simulink library "qlib"  (Simulink 7.0)
libraries: qlib x9, simulink x4
Description:
  | Quaternion Library for Simulink
  |   Version 1.5 (JASP) 20-Jul-2009
  |   ========================================================================
  |   Copyright (c) 2000-2009, Jay A. St. Pierre.  All rights reserved.
  |   This software is licensed under the terms of the BSD license.
  |   See the file license.txt that came with the software for more details.
  |   ========================================================================
  | 
  |   This is a library of blocks that allows manipulation of quaternions.
  | 
  |   The available blocks are:
  | 
  |     Quaternion Normalize
  |     Quaternion Conjugate
  |     Quaternion Multiply
  | 
  |     Quaternion Propagation
  |     Quaternion Vector Transform
  |     Quaternion Vector Rotation
  | 
  |     Quaternion Decomposition
  |     Quaternion to DCM
  |     DCM to Quaternion
  | 
  |   For purposes of this library, a quaternion, q, is just a four element
  |   vector where q(1:3) is the "imaginary" or "vector" portion of the
  |   hypercomplex number, and q(4) is the "real" or "scalar" portion.
  |   Consequently, if q represents a rotation, then:
  | 
  |     q(1) = v1*sin(phi/2)
  |     q(2) = v2*sin(phi/2)
  |     q(3) = v3*sin(phi/2)
  |     q(4) =    cos(phi/2)
  | 
  |   where phi is the amount of rotation about the unit vector [v1 v2 v3].
  | 
  |   IMPORTANT NOTE: For purposes of quaternion/DCM equivalence, the
  |   relationship is chosen to be:
  | 
  |      R v = q* v q
  | 
  |   Therefore a "transform" is (q* v q) and a "rotation" is (q v q*). This
  |   follows the convention used in "Spacecraft Attitude Determination and
  |   Control", edited by James R. Wertz, Copyright 1978.  Note that many
  |   recent uses of quaternions choose the opposite convention (the "left"
  |   quaternion being the equivalent), including many computer graphics
  |   libraries.
  | 
  |   See also QUATERNIONS, the quaternion manipulation toolbox for the
  |   MATLAB command line.  RM2MAT and MAT2RM are also useful for handling
  |   row-major form matrices, and can be found in the Matrix Library for
  |   Simulink.
settings Model: Creator=stpierre  LastModifiedBy=stpierre  ExtModeAutoUpdateStatusClock=off

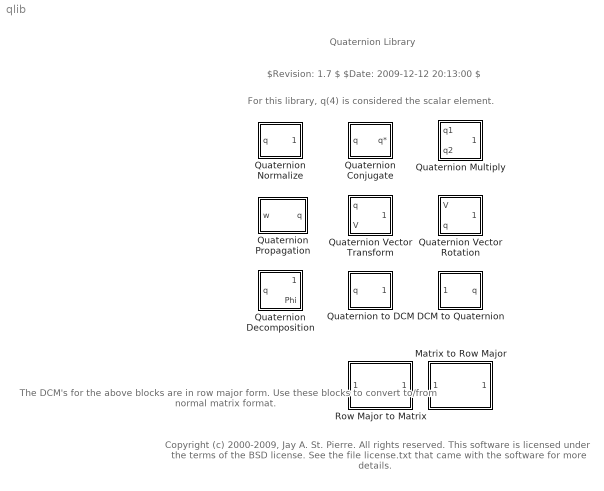
== system qlib ==
  note: Quaternion Library
  note: $Revision: 1.7 $
      | $Date: 2009-12-12 20:13:00 $
  note: For this library, q(4) is considered the scalar element.
  note: Copyright (c) 2000-2009, Jay A. St. Pierre.  All rights reserved.
      | This software is licensed under the terms of the BSD license.
      | See the file license.txt that came with the software for more details.
  note: The DCM's for the
      | above blocks are in
      | row major form.  Use
      | these blocks to convert
      | to/from normal matrix
      | format.
  DCM to Quaternion : Subsystem
      mask Type: DCM to Quaternion
      mask Description:
      | Converts a direction cosine matrix (DCM) to a quaternion that would perform the equivalent vector transformation, i.e., q*vq = Rv, where R is the DCM, v is a vector, and q is the quaternion.
      | 
      | Note that for purposes of quaternion-vector multiplication, a vector is treated as a quaterion with a scalar element of zero.
  Matrix to Row Major : Subsystem
      mask Type: Matrix to Row Major
      mask Description: Converts a matrix to row major vector form.
      mask Display: fprintf('Matrix to\nRow Major');
  Quaternion Conjugate : Subsystem
      mask Type: Quaternion Conjugate
      mask Description: q* = [ -q(1)  -q(2)  -q(3)  q(4) ]
      mask Display: disp('q*')
  Quaternion Decomposition : Subsystem
      mask Type: Quaternion Decomposition
      mask Description:
      | Breaks down a quaternion into its unit vector and total rotation angle about that vector.  If the components of the quaternion are denoted:
      | 
      |      q = [ q(1)  q(2)  q(3)  q(4) ]
      | 
      | Then:
      | 
      |      q(1) = v1 sin(phi/2)
      |      q(2) = v2 sin(phi/2)
      |      q(3) = v3 sin(phi/2)
      |      q(4) = cos(phi/2)
      | 
      | Where phi is the amount of rotation about the unit vector [ v1  v2  v3 ].
  Quaternion Multiply : Subsystem
      mask Type: Quaternion Multiply
      mask Description: Multiplies input quaternions: qout = (q1)(q2)
  Quaternion Normalize : Subsystem  mask(Quaternion Normalize){}
      mask help: qout = q/sqrt(q(1)^2+q(2)^2+q(3)^2+q(4)^2)
      mask init:
      | pos = get_param(gcb, 'Position');
      | width = pos(3) - pos(1); height = pos(4) - pos(2);
      | fontsize = get_param(gcb, 'fontsize');
      | if fontsize==-1, scale=1; else scale=fontsize/10; end
      mask Display:
      | text(width/2-scale*3, (height/2+scale*10), 'q')
      | text(width/2-scale*8, (height/2-scale*6), '||q||')
      | plot([width/2-scale*10 width/2+scale*10], height/2*[1 1])
  Quaternion Propagation : Subsystem  mask(Quaternion Propagation){q0=[0 0 0 1]}
      mask help:
      | Integrates dq/dt to propagate a quaternion, where:
      |
      |     dq/dt = (1/2) (q) ([w 0])
      |
      | and the product (q)([w 0]) is calculated as a quaternion multiplication.
      |
      | The input rates, w, are inertial, but written in the body frame coordinates.  The quaternion indicates the orientation of the body frame with respect to the inertial frame.  The initlal quaternion, q0, must be specfied below.
      |
      | The quaternion is renormalized at each iteration.
      mask init:
      | pos = get_param(gcb, 'Position');
      | width = pos(3) - pos(1); height = pos(4) - pos(2);
      | fontsize = get_param(gcb, 'fontsize');
      | if fontsize==-1, scale=1; else scale=fontsize/10; end
      | 
      | t1=-pi/2:(pi/2)/20:0; t2=pi:-(pi/2)/20:(pi/2);
      | x=[cos(t1)  cos(t2)+2]; y=[sin(t1)+1  sin(t2)+4];
      | 
      | ny=0.9*y/max(y)*scale;
      | nx=0.9*x/max(y)*scale;
      | 
      | s=20;
      | sy=s*(ny - max(ny)/2) + height/2;
      | sx=s*nx + width/2 - 15*scale;
      | 
      | t=0:2*pi/100:2*pi;
      | a=1;
      | tx=a*cos(t)+width/2-5*scale; ty=a*sin(t)+height/2+4*scale;
      mask Display:
      | plot(sx,sy);
      | text(width/2-7*scale, height/2, 'q dt');
      | plot(tx,ty)
  Quaternion Vector Rotation : Subsystem
      mask Type: Quaternion Vector Rotation
      mask Description:
      | Rotates a vector using a quaternion:
      | 
      |     vout = (q)(v)(q*)
      | 
      | The first input is the vector, the second input is the quaternion.
      | 
      | Note that for purposes of quaternion-vector multiplication, a vector is treated as a quaterion with a scalar element of zero.
  Quaternion Vector Transform : Subsystem
      mask Type: Quaternion Vector Transform
      mask Description:
      | Transforms a vector using a quaternion:
      | 
      |     vout = (q*)(v)(q)
      | 
      | The first input is the quaternion, the second input is the vector.
      | 
      | Note that for purposes of quaternion-vector multiplication, a vector is treated as a quaterion with a scalar element of zero.
  Quaternion to DCM : Subsystem
      mask Type: Quaternion to DCM
      mask Description:
      | Converts a quaternion to the direction cosine matrix (DCM) that would perform the equivalent vector transformation, i.e., Rv = q*vq, where R is the DCM, v is a vector, and q is the quaternion.
      | 
      | Note that for purposes of quaternion-vector multiplication, a vector is treated as a quaterion with a scalar element of zero.
  Row Major to Matrix : Subsystem  mask(Row Major to Matrix){rows=3, columns=3}
      mask help: Converts a row major representation of a matrix to a normal matrix.
      mask Display:
      | fprintf('Row Major\nto Matrix\n')
      | text(1, 0, ...
      |     sprintf('%dx%d', rows, columns), ...
      |     'HorizontalAlignment', 'Right', ...
      |     'VerticalAlignment', 'Bottom');

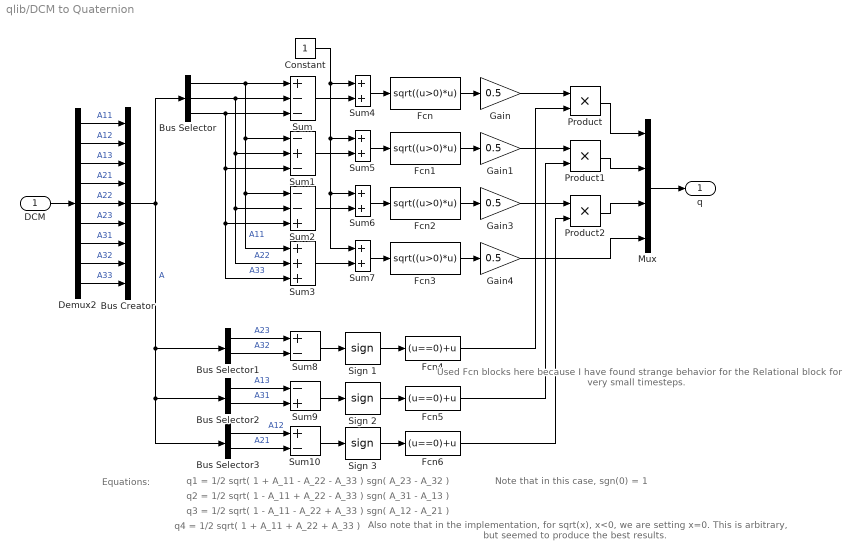
== system qlib/DCM to Quaternion ==
  note: Used Fcn blocks here because
      | I have found strange behavior
      | for the Relational block for
      | very small timesteps.
  note: q1 = 1/2 sqrt( 1 + A_11 - A_22 - A_33 ) sgn( A_23 - A_32 )
  note: q2 = 1/2 sqrt( 1 - A_11 + A_22 - A_33 ) sgn( A_31 - A_13 )
  note: q3 = 1/2 sqrt( 1 - A_11 - A_22 + A_33 ) sgn( A_12 - A_21 )
  note: q4 = 1/2 sqrt( 1 + A_11 + A_22 + A_33 )
  note: Equations:
  note: Note that in this case, sgn(0) = 1
  note: Also note that in the implementation,
      | for sqrt(x), x<0, we are setting x=0.
      | This is arbitrary, but seemed to produce
      | the best results.
  DCM : Inport  PortDimensions=9
  Bus Creator : BusCreator  Inputs=9
  Bus Selector : BusSelector  OutputSignals=A11,A22,A33
  Bus Selector1 : BusSelector  OutputSignals=A23,A32
  Bus Selector2 : BusSelector  OutputSignals=A13,A31
  Bus Selector3 : BusSelector  OutputSignals=A12,A21
  Constant : Constant
  Demux2 : Demux  Outputs=9
  Fcn{,1..3} (4 alike) : Fcn  Expr=sqrt((u>0)*u)
  Fcn4 : Fcn  Expr=(u==0)+u
  Fcn5 : Fcn  Expr=(u==0)+u
  Fcn6 : Fcn  Expr=(u==0)+u
  Gain{,1,3..4} (4 alike) : Gain  Gain=0.5  SaturateOnIntegerOverflow=on
  Mux : Mux
  Product : Product  SaturateOnIntegerOverflow=on  RndMeth=Zero  InputSameDT=on
  Product1 : Product  SaturateOnIntegerOverflow=on  RndMeth=Zero  InputSameDT=on
  Product2 : Product  SaturateOnIntegerOverflow=on  RndMeth=Zero  InputSameDT=on
  Sign 1 : Signum
  Sign 2 : Signum
  Sign 3 : Signum
  Sum : Sum  Inputs=+--  SaturateOnIntegerOverflow=on  InputSameDT=on
  Sum1 : Sum  Inputs=-+-  SaturateOnIntegerOverflow=on  InputSameDT=on
  Sum10 : Sum  Inputs=+-  SaturateOnIntegerOverflow=on  InputSameDT=on
  Sum2 : Sum  Inputs=--+  SaturateOnIntegerOverflow=on  InputSameDT=on
  Sum3 : Sum  Inputs=+++  SaturateOnIntegerOverflow=on  InputSameDT=on
  Sum{4..7} (4 alike) : Sum  SaturateOnIntegerOverflow=on  InputSameDT=on
  Sum8 : Sum  Inputs=+-  SaturateOnIntegerOverflow=on  InputSameDT=on
  Sum9 : Sum  Inputs=-+  SaturateOnIntegerOverflow=on  InputSameDT=on
  q : Outport  InitialOutput=[0 0 0 1]
  wires:
  Sum/1 -> Sum4/2
  Sum1/1 -> Sum5/2
  Constant/1 -> Sum4/1, Sum5/1, Sum6/1, Sum7/1
  Sum4/1 -> Fcn/1
  Sum3/1 -> Sum7/2
  Sum2/1 -> Sum6/2
  Gain/1 -> Product/1
  Gain1/1 -> Product1/1
  Gain3/1 -> Product2/1
  Sum5/1 -> Fcn1/1
  Sum6/1 -> Fcn2/1
  Sum7/1 -> Fcn3/1
  Fcn/1 -> Gain/1
  Fcn1/1 -> Gain1/1
  Fcn3/1 -> Gain4/1
  Fcn2/1 -> Gain3/1
  Sum8/1 -> Sign 1/1
  Fcn4/1 -> Product/2
  Sign 1/1 -> Fcn4/1
  Sum9/1 -> Sign 2/1
  Fcn5/1 -> Product1/2
  Sign 2/1 -> Fcn5/1
  Sum10/1 -> Sign 3/1
  Fcn6/1 -> Product2/2
  Sign 3/1 -> Fcn6/1
  Bus Selector1/1 -> Sum8/1  "A23"
  Bus Selector1/2 -> Sum8/2  "A32"
  Bus Selector/2 -> Sum/2, Sum1/2, Sum3/2, Sum2/2  "A22"
  Bus Selector/1 -> Sum/1, Sum1/1, Sum2/1, Sum3/1  "A11"
  Bus Selector/3 -> Sum/3, Sum1/3, Sum3/3, Sum2/3  "A33"
  Bus Selector2/1 -> Sum9/1  "A13"
  Bus Selector2/2 -> Sum9/2  "A31"
  Bus Selector3/2 -> Sum10/2  "A21"
  Bus Selector3/1 -> Sum10/1  "A12"
  Demux2/1 -> Bus Creator/1  "A11"
  Demux2/2 -> Bus Creator/2  "A12"
  Demux2/3 -> Bus Creator/3  "A13"
  Demux2/4 -> Bus Creator/4  "A21"
  Demux2/5 -> Bus Creator/5  "A22"
  Demux2/6 -> Bus Creator/6  "A23"
  Demux2/7 -> Bus Creator/7  "A31"
  Demux2/8 -> Bus Creator/8  "A32"
  Demux2/9 -> Bus Creator/9  "A33"
  DCM/1 -> Demux2/1
  Bus Creator/1 -> Bus Selector/1, Bus Selector1/1, Bus Selector2/1, Bus Selector3/1  "A"
  Product/1 -> Mux/1
  Product1/1 -> Mux/2
  Product2/1 -> Mux/3
  Gain4/1 -> Mux/4
  Mux/1 -> q/1

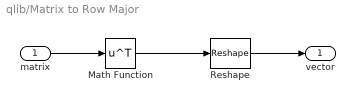
== system qlib/Matrix to Row Major ==
  matrix : Inport
  Math Function : Math  Operator=transpose  OutDataType=sfix(16)  OutScaling=2^0  SaturateOnIntegerOverflow=on
      settings: AttributesFormatString=%<Operator>
  Reshape : Reshape  OutputDimensions=[3, 3]
      settings: AttributesFormatString=Output: %<OutputDimensionality>
  vector : Outport
  wires:
  Math Function/1 -> Reshape/1
  matrix/1 -> Math Function/1
  Reshape/1 -> vector/1

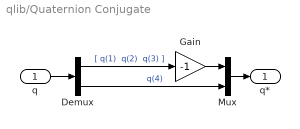
== system qlib/Quaternion Conjugate ==
  q : Inport  PortDimensions=4
  Demux : Demux  Outputs=[3 1]
  Gain : Gain  Gain=-1  SaturateOnIntegerOverflow=on
  Mux : Mux  Inputs=2
  q* : Outport  InitialOutput=0
  wires:
  q/1 -> Demux/1
  Demux/1 -> Gain/1  "[ q(1)  q(2)  q(3) ]"
  Gain/1 -> Mux/1
  Demux/2 -> Mux/2  "q(4)"
  Mux/1 -> q*/1

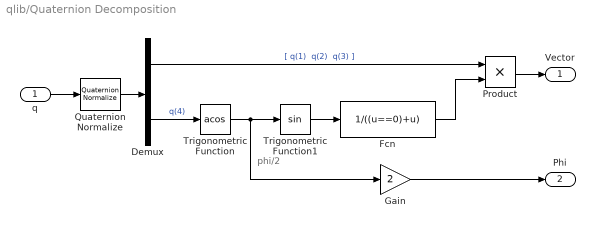
== system qlib/Quaternion Decomposition ==
  note: phi/2
  q : Inport  PortDimensions=4
  Demux : Demux  Outputs=[3 1]
  Fcn : Fcn  Expr=1/((u==0)+u)
  Gain : Gain  Gain=2  SaturateOnIntegerOverflow=on
  Product : Product  SaturateOnIntegerOverflow=on  RndMeth=Zero  InputSameDT=on
  Quaternion Normalize : qlib/Quaternion Normalize
  Trigonometric Function : Trigonometry  Operator=acos
  Trigonometric Function1 : Trigonometry
  Vector : Outport  InitialOutput=0
  Phi : Outport  Port=2  InitialOutput=0
  wires:
  Quaternion Normalize/1 -> Demux/1
  Demux/1 -> Product/1  "[ q(1)  q(2)  q(3) ]"
  Demux/2 -> Trigonometric Function/1  "q(4)"
  Trigonometric Function1/1 -> Fcn/1
  Trigonometric Function/1 -> Trigonometric Function1/1, Gain/1
  Gain/1 -> Phi/1
  q/1 -> Quaternion Normalize/1
  Product/1 -> Vector/1
  Fcn/1 -> Product/2

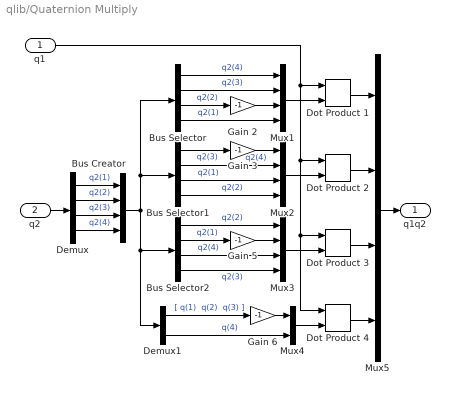
== system qlib/Quaternion Multiply ==
  q1 : Inport  PortDimensions=4
  q2 : Inport  Port=2  PortDimensions=4
  Bus Creator : BusCreator
  Bus Selector : BusSelector  OutputSignals=q2(4),q2(3),q2(2),q2(1)
  Bus Selector1 : BusSelector  OutputSignals=q2(3),q2(4),q2(1),q2(2)
  Bus Selector2 : BusSelector  OutputSignals=q2(2),q2(1),q2(4),q2(3)
  Demux : Demux
  Demux1 : Demux  Outputs=[3 1]
  Dot Product {1..4} (4 alike) : simulink/Math Operations/Dot Product  InputSameDT=on  OutDataType=sfix(16)  OutScaling=2^-10  DoSatur=off
  Gain {2..3,5..6} (4 alike) : Gain  Gain=-1  SaturateOnIntegerOverflow=on
  Mux{1..3,5} (4 alike) : Mux
  Mux4 : Mux  Inputs=2
  q1q2 : Outport  InitialOutput=0
  wires:
  Demux1/2 -> Mux4/2  "q(4)"
  Gain 6/1 -> Mux4/1
  Demux1/1 -> Gain 6/1  "[ q(1)  q(2)  q(3) ]"
  Mux4/1 -> Dot Product 4/2
  Bus Selector2/4 -> Mux3/4  "q2(3)"
  Bus Selector2/1 -> Mux3/1  "q2(2)"
  Gain 5/1 -> Mux3/2
  Bus Selector2/2 -> Gain 5/1  "q2(1)"
  Bus Selector1/4 -> Mux2/4  "q2(2)"
  Bus Selector1/3 -> Mux2/3  "q2(1)"
  Gain 3/1 -> Mux2/1
  Bus Selector1/1 -> Gain 3/1  "q2(3)"
  Bus Selector/4 -> Mux1/4  "q2(1)"
  Gain 2/1 -> Mux1/3
  Bus Selector/3 -> Gain 2/1  "q2(2)"
  Bus Selector/2 -> Mux1/2  "q2(3)"
  Bus Selector/1 -> Mux1/1  "q2(4)"
  Bus Selector1/2 -> Mux2/2  "q2(4)"
  Bus Selector2/3 -> Mux3/3  "q2(4)"
  Mux1/1 -> Dot Product 1/2
  Mux2/1 -> Dot Product 2/2
  Mux3/1 -> Dot Product 3/2
  q1/1 -> Dot Product 1/1, Dot Product 2/1, Dot Product 3/1, Dot Product 4/1
  Dot Product 1/1 -> Mux5/1
  Dot Product 3/1 -> Mux5/3
  Dot Product 4/1 -> Mux5/4
  Mux5/1 -> q1q2/1
  Dot Product 2/1 -> Mux5/2
  Bus Creator/1 -> Demux1/1, Bus Selector2/1, Bus Selector/1, Bus Selector1/1
  q2/1 -> Demux/1
  Demux/1 -> Bus Creator/1  "q2(1)"
  Demux/2 -> Bus Creator/2  "q2(2)"
  Demux/3 -> Bus Creator/3  "q2(3)"
  Demux/4 -> Bus Creator/4  "q2(4)"

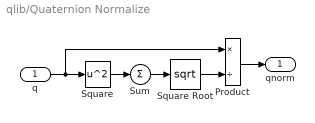
== system qlib/Quaternion Normalize ==
  q : Inport  PortDimensions=4
  Product : Product  Inputs=*/  SaturateOnIntegerOverflow=on  RndMeth=Zero  InputSameDT=on
  Square : Math  Operator=square  SaturateOnIntegerOverflow=on
  Square Root : Math  Operator=sqrt  SaturateOnIntegerOverflow=on
  Sum : Sum  Inputs=1  SaturateOnIntegerOverflow=on  InputSameDT=on
  qnorm : Outport  InitialOutput=0
  wires:
  Product/1 -> qnorm/1
  Square Root/1 -> Product/2
  q/1 -> Product/1, Square/1
  Square/1 -> Sum/1
  Sum/1 -> Square Root/1

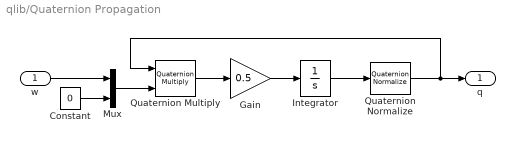
== system qlib/Quaternion Propagation ==
  w : Inport  PortDimensions=3
  Constant : Constant  Value=0
  Gain : Gain  Gain=0.5  SaturateOnIntegerOverflow=on
  Integrator : Integrator  InitialCondition=q0
  Mux : Mux  Inputs=2
  Quaternion Multiply : qlib/Quaternion Multiply
  Quaternion Normalize : qlib/Quaternion Normalize
  q : Outport  InitialOutput=0
  wires:
  Quaternion Multiply/1 -> Gain/1
  Gain/1 -> Integrator/1
  Integrator/1 -> Quaternion Normalize/1
  Quaternion Normalize/1 -> q/1, Quaternion Multiply/1
  w/1 -> Mux/1
  Constant/1 -> Mux/2
  Mux/1 -> Quaternion Multiply/2

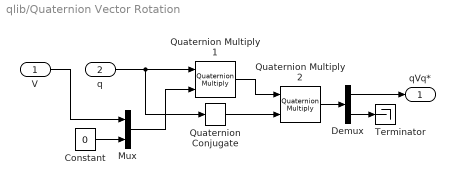
== system qlib/Quaternion Vector Rotation ==
  V : Inport  PortDimensions=3
  q : Inport  Port=2  PortDimensions=4
  Constant : Constant  Value=0
  Demux : Demux  Outputs=[3 1]
  Mux : Mux  Inputs=2
  Quaternion Conjugate : qlib/Quaternion Conjugate
  Quaternion Multiply 1 : qlib/Quaternion Multiply
  Quaternion Multiply 2 : qlib/Quaternion Multiply
  Terminator : Terminator
  qVq* : Outport  InitialOutput=0
  wires:
  q/1 -> Quaternion Conjugate/1, Quaternion Multiply 1/1
  Constant/1 -> Mux/2
  V/1 -> Mux/1
  Demux/1 -> qVq*/1
  Demux/2 -> Terminator/1
  Quaternion Multiply 2/1 -> Demux/1
  Quaternion Multiply 1/1 -> Quaternion Multiply 2/1
  Mux/1 -> Quaternion Multiply 1/2
  Quaternion Conjugate/1 -> Quaternion Multiply 2/2

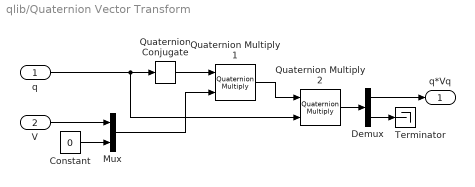
== system qlib/Quaternion Vector Transform ==
  q : Inport  PortDimensions=4
  V : Inport  Port=2  PortDimensions=3
  Constant : Constant  Value=0
  Demux : Demux  Outputs=[3 1]
  Mux : Mux  Inputs=2
  Quaternion Conjugate : qlib/Quaternion Conjugate
  Quaternion Multiply 1 : qlib/Quaternion Multiply
  Quaternion Multiply 2 : qlib/Quaternion Multiply
  Terminator : Terminator
  q*Vq : Outport  InitialOutput=0
  wires:
  V/1 -> Mux/1
  Constant/1 -> Mux/2
  q/1 -> Quaternion Multiply 2/2, Quaternion Conjugate/1
  Quaternion Multiply 2/1 -> Demux/1
  Demux/2 -> Terminator/1
  Demux/1 -> q*Vq/1
  Mux/1 -> Quaternion Multiply 1/2
  Quaternion Conjugate/1 -> Quaternion Multiply 1/1
  Quaternion Multiply 1/1 -> Quaternion Multiply 2/1

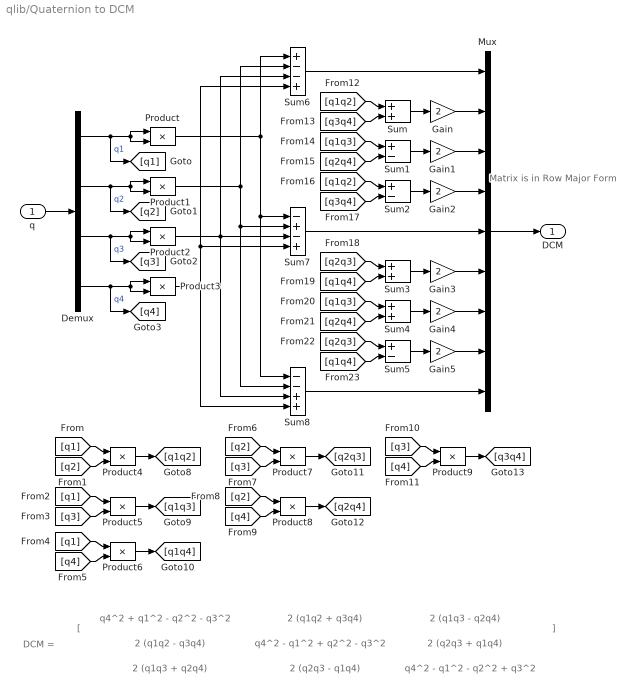
== system qlib/Quaternion to DCM ==
  note: ]
  note: [
  note: Matrix is in
      | Row Major Form
  note: DCM =
  note: 2 (q1q3 + q2q4)
  note: 2 (q1q2 - q3q4)
  note: 2 (q2q3 - q1q4)
  note: 2 (q2q3 + q1q4)
  note: q4^2 - q1^2 - q2^2 + q3^2
  note: q4^2 + q1^2 - q2^2 - q3^2
  note: 2 (q1q3 - q2q4)
  note: 2 (q1q2 + q3q4)
  note: q4^2 - q1^2 + q2^2 - q3^2
  q : Inport  PortDimensions=4
  Demux : Demux
  Gain{,1..5} (6 alike) : Gain  Gain=2  SaturateOnIntegerOverflow=on
  Mux : Mux  Inputs=9
  Product{,1..9} (10 alike) : Product  SaturateOnIntegerOverflow=on  RndMeth=Zero  InputSameDT=on
  Sum : Sum  SaturateOnIntegerOverflow=on  InputSameDT=on
  Sum1 : Sum  Inputs=+-  SaturateOnIntegerOverflow=on  InputSameDT=on
  Sum2 : Sum  Inputs=+-  SaturateOnIntegerOverflow=on  InputSameDT=on
  Sum3 : Sum  SaturateOnIntegerOverflow=on  InputSameDT=on
  Sum4 : Sum  SaturateOnIntegerOverflow=on  InputSameDT=on
  Sum5 : Sum  Inputs=+-  SaturateOnIntegerOverflow=on  InputSameDT=on
  Sum6 : Sum  Inputs=+--+  SaturateOnIntegerOverflow=on  InputSameDT=on
  Sum7 : Sum  Inputs=-+-+  SaturateOnIntegerOverflow=on  InputSameDT=on
  Sum8 : Sum  Inputs=--++  SaturateOnIntegerOverflow=on  InputSameDT=on
  DCM : Outport  InitialOutput=0
  wires:
  Product9/1 -> [q3q4]
  [q4] -> Product9/2
  [q3] -> Product9/1
  Product8/1 -> [q2q4]
  [q4] -> Product8/2
  [q2] -> Product8/1
  Product7/1 -> [q2q3]
  [q3] -> Product7/2
  [q2] -> Product7/1
  Product6/1 -> [q1q4]
  [q4] -> Product6/2
  [q1] -> Product6/1
  Product5/1 -> [q1q3]
  [q3] -> Product5/2
  [q1] -> Product5/1
  Product4/1 -> [q1q2]
  [q2] -> Product4/2
  [q1] -> Product4/1
  q/1 -> Demux/1
  Product3/1 -> Sum8/4, Sum7/4, Sum6/4
  Product2/1 -> Sum8/3, Sum7/3, Sum6/3
  Product1/1 -> Sum8/2, Sum7/2, Sum6/2
  Product/1 -> Sum8/1, Sum7/1, Sum6/1
  Sum8/1 -> Mux/9
  Sum7/1 -> Mux/5
  Sum5/1 -> Gain5/1
  [q2q3] -> Sum5/1
  [q1q4] -> Sum5/2
  Sum4/1 -> Gain4/1
  [q1q3] -> Sum4/1
  [q2q4] -> Sum4/2
  Sum3/1 -> Gain3/1
  [q2q3] -> Sum3/1
  [q1q4] -> Sum3/2
  Sum2/1 -> Gain2/1
  [q1q2] -> Sum2/1
  [q3q4] -> Sum2/2
  Sum1/1 -> Gain1/1
  [q1q3] -> Sum1/1
  [q2q4] -> Sum1/2
  Sum/1 -> Gain/1
  [q1q2] -> Sum/1
  [q3q4] -> Sum/2
  Gain5/1 -> Mux/8
  Gain4/1 -> Mux/7
  Gain3/1 -> Mux/6
  Gain2/1 -> Mux/4
  Mux/1 -> DCM/1
  Demux/1 -> Product/1, Product/2, [q1]  "q1"
  Demux/2 -> Product1/2, Product1/1, [q2]  "q2"
  Demux/3 -> Product2/1, Product2/2, [q3]  "q3"
  Demux/4 -> Product3/2, Product3/1, [q4]  "q4"
  Gain1/1 -> Mux/3
  Gain/1 -> Mux/2
  Sum6/1 -> Mux/1

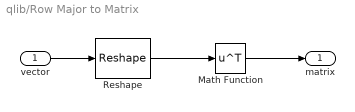
== system qlib/Row Major to Matrix ==
  vector : Inport
  Math Function : Math  Operator=transpose  OutDataType=sfix(16)  OutScaling=2^0  SaturateOnIntegerOverflow=on
      settings: AttributesFormatString=%<Operator>
  Reshape : Reshape  OutputDimensionality=Customize  OutputDimensions=[3, 3]
      settings: AttributesFormatString=Output Dimensions = %<OutputDimensions>
  matrix : Outport
  wires:
  Math Function/1 -> matrix/1
  vector/1 -> Reshape/1
  Reshape/1 -> Math Function/1
